simulink model "Dead_Reckoning"  (R2021a)
settings: Solver=FixedStepDiscrete  StartTime=0.0  StopTime=1150  FixedStep=0.01  RelTol=1e-3
undefined symbols (not defined in the file): t_per_rot, wheelr
libraries: mobileRoboticsTrainingLib x3
settings Model: EnablePacing=on  Creator=DELL  LastModifiedBy=DELL

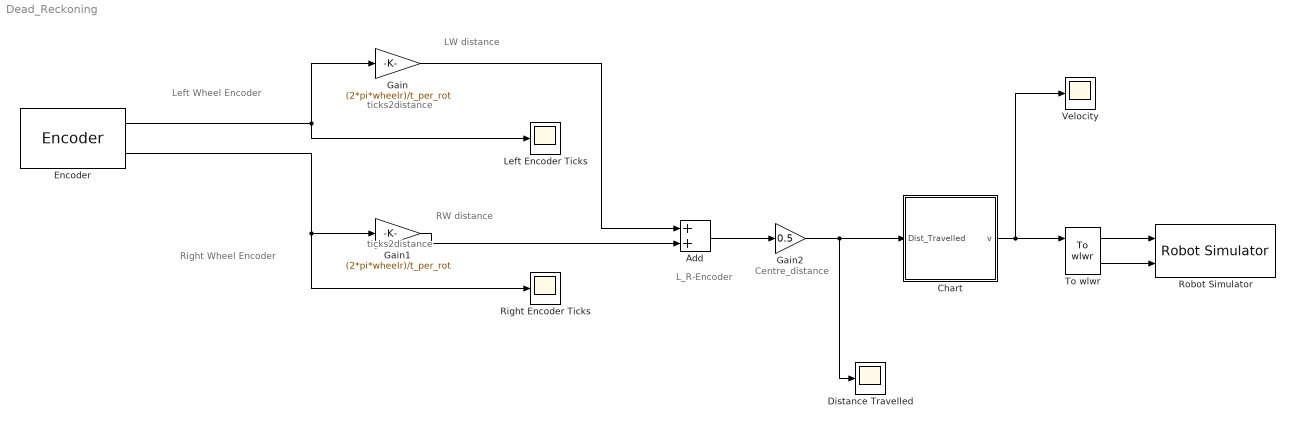
== system Dead_Reckoning ==
  note: Centre_distance
  note: RW distance
  note: L_R-Encoder
  note: ticks2distance
  note: Right Wheel Encoder
  note: LW
      |  distance
  note: ticks2distance
  note: Left Wheel Encoder
  Add : Sum
  Chart : Stateflow chart  TreatAsAtomicUnit=on
  Distance Travelled : Scope
  Encoder : mobileRoboticsTrainingLib/Encoder  axleLength=axleLength  wheelR=wheelr  ticksPerRot=t_per_rot
      settings: SourceProductName=Mobile Robotics Training Library
  Gain : Gain  Gain=(2*pi*wheelr)/t_per_rot
  Gain1 : Gain  Gain=(2*pi*wheelr)/t_per_rot
  Gain2 : Gain  Gain=0.5
  Left Encoder Ticks : Scope
  "Right Encoder Ticks " : Scope
  Robot Simulator : mobileRoboticsTrainingLib/Robot Simulator  Priority=99  mapVar=[]  startX=1  startY=1  startTheta=0  axleLength=axleLength  wheelR=wheelr
  To wlwr : mobileRoboticsTrainingLib/To wlwr  axleLength=axleLength  wheelR=wheelr
  Velocity : Scope
  wires:
  Encoder/1 -> Gain/1, Left Encoder Ticks/1
  Gain/1 -> Add/1
  Encoder/2 -> "Right Encoder Ticks "/1, Gain1/1
  Gain1/1 -> Add/2
  Add/1 -> Gain2/1
  Gain2/1 -> Chart/1(Dist_Travelled), Distance Travelled/1
  Chart/1(v) -> Velocity/1, To wlwr/1
  To wlwr/1 -> Robot Simulator/1
  To wlwr/2 -> Robot Simulator/2

== stateflow chart Dead_Reckoning/Chart ==
  note: %Start
  state MoveForward
    entry: v=0.1
  state Stop
    entry: v=0
  (default) -> MoveForward
  MoveForward -> Stop : [Dist_Travelled>=1]
  data: Dist_Travelled input; v output
